simulink model "project"  (R2020b)
settings: Solver=VariableStepAuto  StartTime=0.0  StopTime=inf  RelTol=1e-3
libraries: simulink x3
settings Model: EnablePacing=on  Creator=99003757  LastModifiedBy=99003757
settings ConfigComp: CovEnable=on  RecordCoverage=on  CovMetricSettings=dcmwe  CovModelRefEnable=on

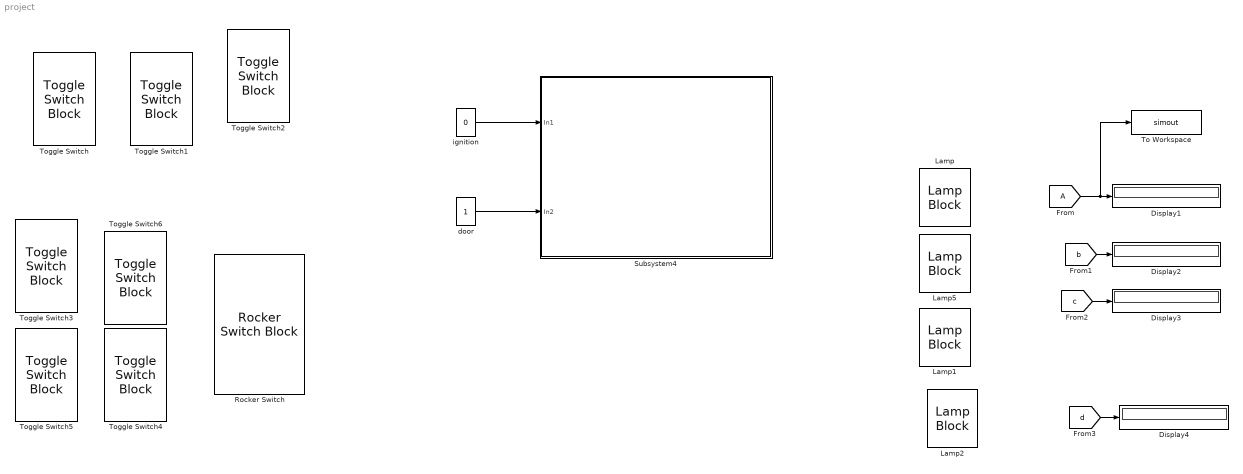
== system project ==
  Display{1..4} (4 alike) : Display
  Lamp{,1..2,5} (4 alike) : LampBlock
  Rocker Switch : RockerSwitchBlock  LabelPosition=Bottom
      settings: Values={{'Off', 'On'}, [2 1]}
  Subsystem4 : Subsystem
  To Workspace : ToWorkspace  VariableName=simout  SaveFormat=Timeseries  SampleTime=-1
  Toggle Switch{,1..6} (7 alike) : ToggleSwitchBlock
  door : Constant
  "ignition " : Constant  Value=0
  wires:
  [A] -> To Workspace/1, Display1/1
  [b] -> Display2/1
  [c] -> Display3/1
  [d] -> Display4/1
  "ignition "/1 -> Subsystem4/1(In1)
  door/1 -> Subsystem4/2(In2)

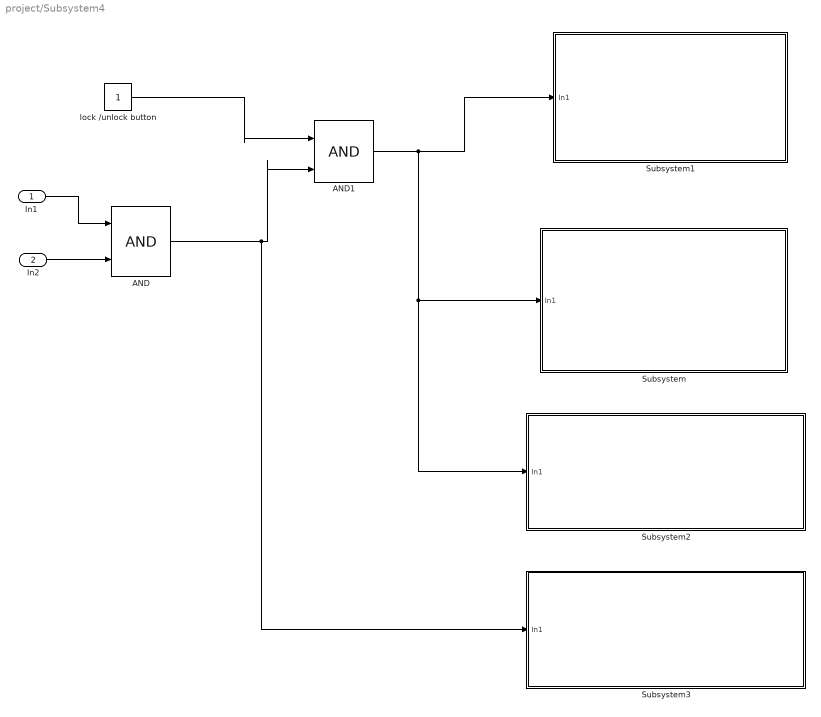
== system project/Subsystem4 ==
  In1 : Inport
  In2 : Inport  Port=2
  AND : Logic  IconShape=distinctive  AllPortsSameDT=off  OutDataTypeStr=boolean
  AND1 : Logic  IconShape=distinctive  AllPortsSameDT=off  OutDataTypeStr=boolean
  Subsystem : Subsystem
  Subsystem1 : Subsystem
  Subsystem2 : Subsystem
  Subsystem3 : Subsystem
  lock /unlock button : Constant
  wires:
  lock /unlock button/1 -> AND1/1
  In2/1 -> AND/2
  In1/1 -> AND/1
  AND1/1 -> Subsystem2/1(In1), Subsystem/1(In1), Subsystem1/1(In1)
  AND/1 -> Subsystem3/1(In1), AND1/2

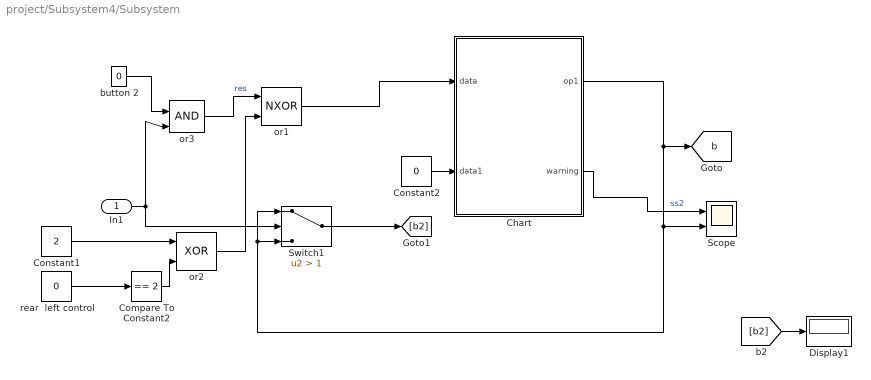
== system project/Subsystem4/Subsystem ==
  In1 : Inport
  Chart : Stateflow chart  TreatAsAtomicUnit=on
  Compare To Constant2 : simulink/Logic and Bit Operations/Compare To Constant  relop===  const=2  OutDataTypeStr=boolean
  Constant1 : Constant  Value=2
  Constant2 : Constant  Value=0
  Display1 : Display
  Scope : Scope  NumInputPorts=2
  Switch1 : Switch  Criteria=u2 > Threshold  Threshold=1
  button 2 : Constant  Value=0
  or1 : Logic  Operator=NXOR  IconShape=distinctive  AllPortsSameDT=off  OutDataTypeStr=boolean
  or2 : Logic  Operator=XOR  IconShape=distinctive  AllPortsSameDT=off  OutDataTypeStr=boolean
  or3 : Logic  IconShape=distinctive  AllPortsSameDT=off  OutDataTypeStr=boolean
  rear  left control : Constant  Value=0
  tag scope: b=global
  wires:
  [b2] -> Display1/1
  button 2/1 -> or3/1
  rear  left control/1 -> Compare To Constant2/1
  Constant1/1 -> or2/1
  Compare To Constant2/1 -> or2/2
  Switch1/1 -> [b2]
  In1/1 -> Switch1/2, or3/2
  Chart/1(op1) -> [b], Switch1/3, Switch1/1, Scope/2
  Constant2/1 -> Chart/2(data1)
  Chart/2(warning) -> Scope/1  "ss2"
  or3/1 -> or1/1  "res"
  or2/1 -> or1/2
  or1/1 -> Chart/1(data)

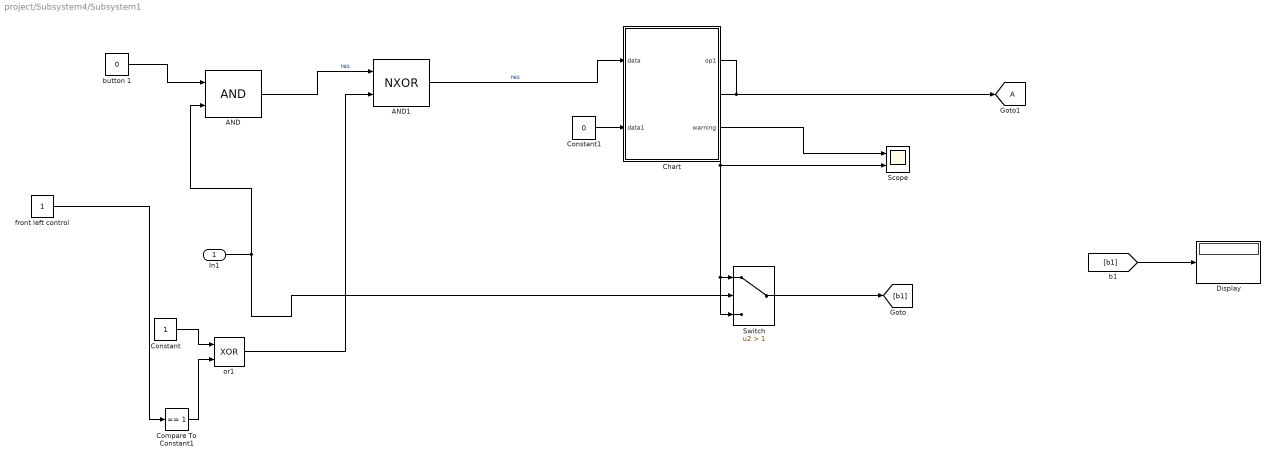
== system project/Subsystem4/Subsystem1 ==
  In1 : Inport
  AND : Logic  IconShape=distinctive  AllPortsSameDT=off  OutDataTypeStr=boolean
  AND1 : Logic  Operator=NXOR  IconShape=distinctive  AllPortsSameDT=off  OutDataTypeStr=boolean
  Chart : Stateflow chart  TreatAsAtomicUnit=on
  Compare To Constant1 : simulink/Logic and Bit Operations/Compare To Constant  relop===  const=1  OutDataTypeStr=boolean
  Constant : Constant
  Constant1 : Constant  Value=0
  Display : Display
  Scope : Scope  NumInputPorts=2
  Switch : Switch  Criteria=u2 > Threshold  Threshold=1
  "button 1 " : Constant  Value=0
  front left control : Constant
  or1 : Logic  Operator=XOR  IconShape=distinctive  AllPortsSameDT=off  OutDataTypeStr=boolean
  tag scope: A=global
  wires:
  In1/1 -> AND/2, Switch/2
  "button 1 "/1 -> AND/1
  Constant/1 -> or1/1
  Switch/1 -> [b1]
  front left control/1 -> Compare To Constant1/1
  Compare To Constant1/1 -> or1/2
  [b1] -> Display/1
  Chart/1(op1) -> Switch/3, Switch/1, Scope/2, [A]
  Chart/2(warning) -> Scope/1
  Constant1/1 -> Chart/2(data1)
  or1/1 -> AND1/2
  AND/1 -> AND1/1  "res"
  AND1/1 -> Chart/1(data)  "res"

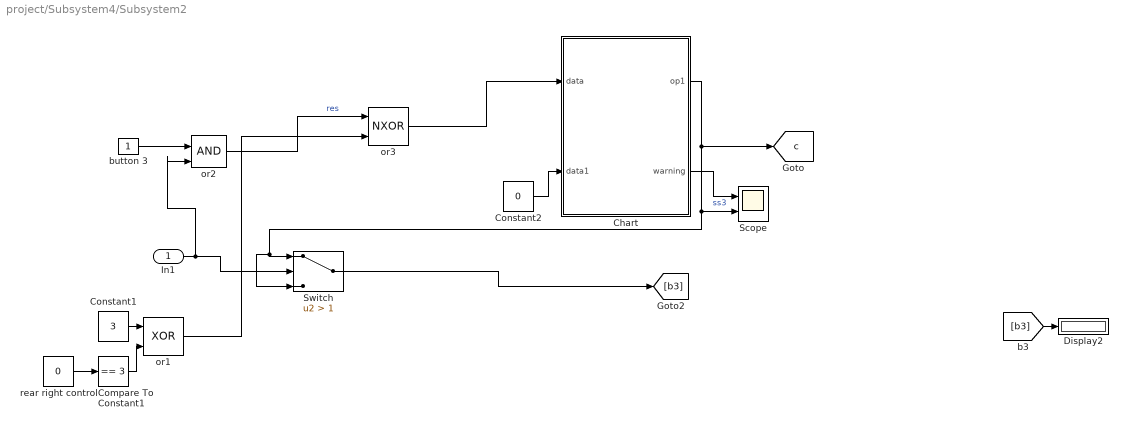
== system project/Subsystem4/Subsystem2 ==
  In1 : Inport
  Chart : Stateflow chart  TreatAsAtomicUnit=on
  Compare To Constant1 : simulink/Logic and Bit Operations/Compare To Constant  relop===  const=3  OutDataTypeStr=boolean
  Constant1 : Constant  Value=3
  Constant2 : Constant  Value=0
  Display2 : Display
  Scope : Scope  NumInputPorts=2
  Switch : Switch  Criteria=u2 > Threshold  Threshold=1
  button 3 : Constant
  or1 : Logic  Operator=XOR  IconShape=distinctive  AllPortsSameDT=off  OutDataTypeStr=boolean
  or2 : Logic  IconShape=distinctive  AllPortsSameDT=off  OutDataTypeStr=boolean
  or3 : Logic  Operator=NXOR  IconShape=distinctive  AllPortsSameDT=off  OutDataTypeStr=boolean
  rear right control : Constant  Value=0
  tag scope: c=global
  wires:
  Constant1/1 -> or1/1
  [b3] -> Display2/1
  Compare To Constant1/1 -> or1/2
  rear right control/1 -> Compare To Constant1/1
  button 3/1 -> or2/1
  Switch/1 -> [b3]
  In1/1 -> or2/2, Switch/2
  Chart/2(warning) -> Scope/1  "ss3"
  Constant2/1 -> Chart/2(data1)
  Chart/1(op1) -> [c], Scope/2, Switch/3, Switch/1
  or1/1 -> or3/2
  or2/1 -> or3/1  "res"
  or3/1 -> Chart/1(data)

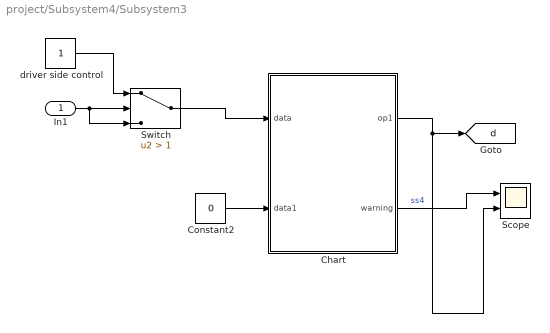
== system project/Subsystem4/Subsystem3 ==
  In1 : Inport
  Chart : Stateflow chart  TreatAsAtomicUnit=on
  Constant2 : Constant  Value=0
  Scope : Scope  NumInputPorts=2
  Switch : Switch  Criteria=u2 > Threshold  Threshold=1
  driver side control : Constant
  tag scope: d=global
  wires:
  Chart/2(warning) -> Scope/1  "ss4"
  Constant2/1 -> Chart/2(data1)
  Chart/1(op1) -> [d], Scope/2
  In1/1 -> Switch/3, Switch/2
  driver side control/1 -> Switch/1
  Switch/1 -> Chart/1(data)

== stateflow chart project/Subsystem4/Subsystem/Chart ==
  state Normal
    state Start
      entry:
      op1 = 25;
    state second
      entry:
      op1 = 100;
    state PrepareToStop
      entry:
      op1 = 75;
    state Go
      % Green light
      entry:
      op1 = 50;
    (default) -> Start
    Start -> (junction 9)
    (junction 9) -> (junction 6) : after(3,sec)
    PrepareToStop -> second : after(3,sec)
    (junction 6) -> Go
    Go -> PrepareToStop : after(3,sec)
  state Fault
    entry:
    op1 =0;
    state BlinkOn
      % Red light
      entry:
      warning = 1;
    (default) -> BlinkOn
  state block_start
    entry:
  state Normal2
    state state5
      entry:
      op1=0
    state Start1
      entry:
      op1=op1;
    state two
      entry:
      op1 = 0;
    state four3
      entry:
      op1 = 0;
    state three
      entry:
      op1 = 25;
    state three1
      entry:
      op1 = 0;
    state five2
      entry:
      op1=0;
    state five
      entry:
      op1=50;
    state five1
      entry:
      op1=25;
    state four2
      entry:
      op1 = 25;
    state four
      entry:
      op1 = 75;
    state four1
      entry:
      op1 = 50;
    Start1 -> state5 [order 4] : [op1==0]
    (default) -> Start1
    Start1 -> (junction 142) [order 2] : after(1,sec)[op1==25]
    (junction 142) -> four3
    Start1 -> (junction 89) [order 3]
    Start1 -> (junction 103) [order 5]
    Start1 -> (junction 48) [order 1]
    (junction 103) -> (junction 104) : after(3,sec)[op1==50]
    (junction 48) -> (junction 49) : after(3,sec)[op1==100]
    (junction 89) -> (junction 90) : after(3,sec)[op1==75]
    three -> two : after(3,sec)[op1==25]
    (junction 104) -> four2
    (junction 49) -> four
    five -> three : after(3,sec)[op1==50]
    (junction 90) -> four1
    five1 -> three1 : after(3,sec)[op1==25]
    four2 -> five2 : after(3,sec)[op1==25]
    four -> five : after(3,sec)[op1==75]
    four1 -> five1 : after(3,sec)[op1==50]
  (default) -> block_start
  block_start -> Normal2 [order 2] : [data == 0]
  Normal -> Fault [order 1] : [data1 == 1]
  block_start -> Normal [order 1] : [data ==1]
  Normal2 -> block_start [order 1] : [data ==1]
  Normal -> block_start [order 2] : [data ==0]
  Fault -> Normal [order 1] : [data1 == 0]
  Fault -> Normal2 [order 2] : [data1 ==0]
  Normal2 -> Fault [order 2] : [data1==1]
  data: data input; data1 input; op1 output =0; warning output

== stateflow chart project/Subsystem4/Subsystem2/Chart ==
  state Normal
    state Start
      entry:
      op1 = 25;
    state second
      entry:
      op1 = 100;
    state PrepareToStop
      entry:
      op1 = 75;
    state Go
      % Green light
      entry:
      op1 = 50;
    (default) -> Start
    Start -> (junction 9)
    (junction 9) -> (junction 6) : after(3,sec)
    PrepareToStop -> second : after(3,sec)
    (junction 6) -> Go
    Go -> PrepareToStop : after(3,sec)
  state Fault
    entry:
    op1 =0;
    state BlinkOn
      % Red light
      entry:
      warning = 1;
    (default) -> BlinkOn
  state block_start
    entry:
  state Normal2
    state state5
      entry:
      op1=0
    state Start1
      entry:
    state two
      entry:
      op1 = 0;
    state four3
      entry:
      op1 = 0;
    state three
      entry:
      op1 = 25;
    state three1
      entry:
      op1 = 0;
    state five2
      entry:
      op1=0;
    state five
      entry:
      op1=50;
    state five1
      entry:
      op1=25;
    state four2
      entry:
      op1 = 25;
    state four
      entry:
      op1 = 75;
    state four1
      entry:
      op1 = 50;
    Start1 -> state5 [order 2] : [op1==0]
    (default) -> Start1
    Start1 -> (junction 143) [order 3] : after(1,sec)[op1==25]
    (junction 143) -> four3
    Start1 -> (junction 89) [order 4]
    Start1 -> (junction 103) [order 5]
    Start1 -> (junction 48) [order 1]
    (junction 103) -> (junction 104) : after(3,sec)[op1==50]
    (junction 48) -> (junction 49) : after(3,sec)[op1==100]
    (junction 89) -> (junction 90) : after(3,sec)[op1==75]
    three -> two : after(3,sec)[op1==25]
    (junction 104) -> four2
    (junction 49) -> four
    five -> three : after(3,sec)[op1==50]
    (junction 90) -> four1
    five1 -> three1 : after(3,sec)[op1==25]
    four2 -> five2 : after(3,sec)[op1==25]
    four -> five : after(3,sec)[op1==75]
    four1 -> five1 : after(3,sec)[op1==50]
  (default) -> block_start
  block_start -> Normal2 [order 2] : [data == 0]
  Normal -> Fault [order 1] : [data1 == 1]
  block_start -> Normal [order 1] : [data ==1]
  Normal2 -> block_start [order 1] : [data ==1]
  Normal -> block_start [order 2] : [data ==0]
  Fault -> Normal [order 1] : [data1 == 0]
  Fault -> Normal2 [order 2] : [data1 ==0]
  Normal2 -> Fault [order 2] : [data1==1]
  data: data input; data1 input; op1 output =0; warning output

== stateflow chart project/Subsystem4/Subsystem1/Chart ==
  state Normal
    state Start
      entry:
      op1 = 25;
    state second
      entry:
      op1 = 100;
    state PrepareToStop
      entry:
      op1 = 75;
    state Go
      % Green light
      entry:
      op1 = 50;
    (default) -> Start
    Start -> (junction 9)
    (junction 9) -> (junction 6) : after(3,sec)
    PrepareToStop -> second : after(3,sec)
    (junction 6) -> Go
    Go -> PrepareToStop : after(3,sec)
  state Fault
    entry:
    op1 =0;
    state BlinkOn
      % Red light
      entry:
      warning = 1;
    (default) -> BlinkOn
  state block_start
    entry:
  state Normal2
    state state5
      entry:
      op1=0
    state Start1
      entry:
      op1=op1;
    state two
      entry:
      op1 = 0;
    state four3
      entry:
      op1 = 0;
    state three
      entry:
      op1 = 25;
    state three1
      entry:
      op1 = 0;
    state five2
      entry:
      op1=0;
    state five
      entry:
      op1=50;
    state five1
      entry:
      op1=25;
    state four2
      entry:
      op1 = 25;
    state four
      entry:
      op1 = 75;
    state four1
      entry:
      op1 = 50;
    Start1 -> state5 [order 4] : [op1==0]
    (default) -> Start1
    Start1 -> (junction 143) [order 2] : after(1,sec)[op1==25]
    (junction 143) -> four3
    Start1 -> (junction 89) [order 3]
    Start1 -> (junction 103) [order 5]
    Start1 -> (junction 48) [order 1]
    (junction 103) -> (junction 104) : after(3,sec)[op1==50]
    (junction 48) -> (junction 49) : after(3,sec)[op1==100]
    (junction 89) -> (junction 90) : after(3,sec)[op1==75]
    three -> two : after(3,sec)[op1==25]
    (junction 104) -> four2
    (junction 49) -> four
    five -> three : after(3,sec)[op1==50]
    (junction 90) -> four1
    five1 -> three1 : after(3,sec)[op1==25]
    four2 -> five2 : after(3,sec)[op1==25]
    four -> five : after(3,sec)[op1==75]
    four1 -> five1 : after(3,sec)[op1==50]
  (default) -> block_start
  block_start -> Normal2 [order 2] : [data == 0]
  Normal -> Fault [order 1] : [data1 == 1]
  block_start -> Normal [order 1] : [data ==1 ]
  Normal2 -> block_start [order 1] : [data ==1]
  Normal -> block_start [order 2] : [data == 0]
  Fault -> Normal [order 1] : [data1 == 0]
  Fault -> Normal2 [order 2] : [data1 ==0]
  Normal2 -> Fault [order 2] : [data1==1]
  data: data input; data1 input; op1 output =0; warning output

== stateflow chart project/Subsystem4/Subsystem3/Chart ==
  state Normal
    state Start
      entry:
      op1 = 25;
    state second
      entry:
      op1 = 100;
    state PrepareToStop
      entry:
      op1 = 75;
    state Go
      % Green light
      entry:
      op1 = 50;
    (default) -> Start
    Start -> (junction 9)
    (junction 9) -> (junction 6) : after(3,sec)
    PrepareToStop -> second : after(3,sec)
    (junction 6) -> Go
    Go -> PrepareToStop : after(3,sec)
  state Fault
    entry:
    op1 =0;
    state BlinkOn
      % Red light
      entry:
      warning = 1;
    (default) -> BlinkOn
  state block_start
    entry:
  state Normal2
    state state5
      entry:
      op1=0
    state Start1
      entry:
      op1=op1;
    state two
      entry:
      op1 = 0;
    state four3
      entry:
      op1 = 0;
    state three
      entry:
      op1 = 25;
    state three1
      entry:
      op1 = 0;
    state five2
      entry:
      op1=0;
    state five
      entry:
      op1=50;
    state five1
      entry:
      op1=25;
    state four2
      entry:
      op1 = 25;
    state four
      entry:
      op1 = 75;
    state four1
      entry:
      op1 = 50;
    Start1 -> state5 [order 4] : [op1==0]
    (default) -> Start1
    Start1 -> (junction 142) [order 2] : after(1,sec)[op1==25]
    Start1 -> (junction 89) [order 3]
    Start1 -> (junction 103) [order 5]
    (junction 142) -> four3
    Start1 -> (junction 48) [order 1]
    (junction 103) -> (junction 104) : after(3,sec)[op1==50]
    (junction 48) -> (junction 49) : after(3,sec)[op1==100]
    (junction 89) -> (junction 90) : after(3,sec)[op1==75]
    three -> two : after(3,sec)[op1==25]
    (junction 104) -> four2
    (junction 49) -> four
    five -> three : after(3,sec)[op1==50]
    (junction 90) -> four1
    five1 -> three1 : after(3,sec)[op1==25]
    four2 -> five2 : after(3,sec)[op1==25]
    four -> five : after(3,sec)[op1==75]
    four1 -> five1 : after(3,sec)[op1==50]
  (default) -> block_start
  block_start -> Normal2 [order 2] : [data == 0]
  Normal -> Fault [order 1] : [data1 == 1]
  block_start -> Normal [order 1] : [data ==1]
  Normal2 -> block_start [order 1] : [data ==1]
  Normal -> block_start [order 2] : [data ==0]
  Fault -> Normal [order 1] : [data1 == 0]
  Fault -> Normal2 [order 2] : [data1 ==0]
  Normal2 -> Fault [order 2] : [data1==1]
  data: data input; data1 input; op1 output =0; warning output
